simulink model "example_sdofplant"  (R2024b)
settings: Solver=FixedStepAuto  StartTime=0  StopTime=200  FixedStep=5/1000  RelTol=1e-3
model workspace (MAT data in the model file):
  Sig : Simulink.Signal (value not decoded)
  Sig1 : Simulink.Signal (value not decoded)
  Sig2 : Simulink.Signal (value not decoded)
  Sig3 : Simulink.Signal (value not decoded)
  Sig4 : Simulink.Signal (value not decoded)
  Sig5 : Simulink.Signal (value not decoded)
  Sig6 : Simulink.Signal (value not decoded)
values from neighbouring files (symbols this model uses):
  aerody =     [vtol50kg_airframe_data.mat]    (also in vtol50kg_airframe_init.m = init_aerody; vtol50kg_initdata.m = init_aerody)
  engine =     [vtol50kg_airframe_data.mat]    (also in vtol50kg_airframe_init.m = init_engine; vtol50kg_initdata.m = init_engine)
  mass =     [vtol50kg_airframe_data.mat]    (also in vtol50kg_airframe_init.m = init_weight; vtol50kg_initdata.m = init_weight)
  motor =     [vtol50kg_airframe_data.mat]    (also in vtol50kg_airframe_init.m = init_motor; vtol50kg_initdata.m = init_motor)
undefined symbols (not defined in the file or in its folder): convertTo, datetime, Earth, F, Light, MIL, plant, WGS84, WMM2020
libraries: aerolibconvert2 x5, aerolibasang x5, aerolibwind2 x3, aerolibactuator x2, shared6dof x1, aerolibatmos2 x1, aerolibtransform2 x1, aerolibgravity2 x1
(part 2 of 2)

== system example_sdofplant/state/Variant Subsystem/Subsystem1 ==
  h(m) : Inport
  μ(deg) : Inport  Port=2
  l(deg) : Inport  Port=3
  World Magnetic Model : aerolibgravity2/World Magnetic Model  model=WMM2020 (2020-2025)  customFile='WMM2020.COF'  units=Metric (MKS)  time_in=off  month=January  day=1  year=2020  action=Error  h_out=on  dec_out=on  inc_out=on  ti_out=on
  XYZ(nT) : Outport
  H(nT) : Outport  Port=2
  D(deg) : Outport  Port=3
  I(deg) : Outport  Port=4
  F(nT) : Outport  Port=5
  wires:
  h(m)/1 -> World Magnetic Model/1
  World Magnetic Model/1 -> XYZ(nT)/1
  World Magnetic Model/2 -> H(nT)/1
  World Magnetic Model/3 -> D(deg)/1
  World Magnetic Model/4 -> I(deg)/1
  World Magnetic Model/5 -> F(nT)/1
  l(deg)/1 -> World Magnetic Model/3
  μ(deg)/1 -> World Magnetic Model/2

== system example_sdofplant/actuator/fixed wing/actuator dyanmics/Variant Subsystem ==
  note: 1) Add Subsystem or Model blocks as valid variant choices.
      | 2) You cannot connect blocks at this level. At simulation, connectivity is automatically
      | determined, based on the active variant and port name matching.
  In1 : Inport
  Subsystem : Subsystem  VariantControl=true
  Subsystem1 : Subsystem  VariantControl=false
  Out1 : Outport

== system example_sdofplant/actuator/fixed wing/aerodynamics/basic ==
  alpha : Inport  Unit=deg
  beta : Inport  Port=2  Unit=deg
  2-D Lookup Table : Lookup_n-D  LookupTableObject=''  BreakpointsForDimension1=aerody.basic.cx.alpha  BreakpointsForDimension2=aerody.basic.cx.beta  BreakpointsForDimension1FirstPoint=10  BreakpointsForDimension2FirstPoint=10  BreakpointsForDimension1Spacing=12  BreakpointsForDimension2Spacing=12  IndexSearchMethod=Linear search  BeginIndexSearchUsingPreviousIndexResult=on  Table=aerody.basic.cx.coeff  ExtrapMethod=Clip  DiagnosticForOutOfRangeInput=Warning  InternalRulePriority=Speed  RndMeth=Simplest
      settings: InputPortMap=u0,u1
  2-D Lookup Table1 : Lookup_n-D  LookupTableObject=''  BreakpointsForDimension1=aerody.basic.cy.alpha  BreakpointsForDimension2=aerody.basic.cy.beta  BreakpointsForDimension1FirstPoint=10  BreakpointsForDimension2FirstPoint=10  BreakpointsForDimension1Spacing=12  BreakpointsForDimension2Spacing=12  IndexSearchMethod=Linear search  BeginIndexSearchUsingPreviousIndexResult=on  Table=aerody.basic.cy.coeff  ExtrapMethod=Clip  DiagnosticForOutOfRangeInput=Warning  InternalRulePriority=Speed  RndMeth=Simplest
      settings: InputPortMap=u0,u1
  2-D Lookup Table2 : Lookup_n-D  LookupTableObject=''  BreakpointsForDimension1=aerody.basic.cz.alpha  BreakpointsForDimension2=aerody.basic.cz.beta  BreakpointsForDimension1FirstPoint=10  BreakpointsForDimension2FirstPoint=10  BreakpointsForDimension1Spacing=12  BreakpointsForDimension2Spacing=12  IndexSearchMethod=Linear search  BeginIndexSearchUsingPreviousIndexResult=on  Table=aerody.basic.cz.coeff  ExtrapMethod=Clip  DiagnosticForOutOfRangeInput=Warning  InternalRulePriority=Speed  RndMeth=Simplest
      settings: InputPortMap=u0,u1
  2-D Lookup Table3 : Lookup_n-D  LookupTableObject=''  BreakpointsForDimension1=aerody.basic.cll.alpha  BreakpointsForDimension2=aerody.basic.cll.beta  BreakpointsForDimension1FirstPoint=10  BreakpointsForDimension2FirstPoint=10  BreakpointsForDimension1Spacing=12  BreakpointsForDimension2Spacing=12  IndexSearchMethod=Linear search  BeginIndexSearchUsingPreviousIndexResult=on  Table=aerody.basic.cll.coeff  ExtrapMethod=Clip  DiagnosticForOutOfRangeInput=Warning  InternalRulePriority=Speed  RndMeth=Simplest
      settings: InputPortMap=u0,u1
  2-D Lookup Table4 : Lookup_n-D  LookupTableObject=''  BreakpointsForDimension1=aerody.basic.cm.alpha  BreakpointsForDimension2=aerody.basic.cm.beta  BreakpointsForDimension1FirstPoint=10  BreakpointsForDimension2FirstPoint=10  BreakpointsForDimension1Spacing=12  BreakpointsForDimension2Spacing=12  IndexSearchMethod=Linear search  BeginIndexSearchUsingPreviousIndexResult=on  Table=aerody.basic.cm.coeff  ExtrapMethod=Clip  DiagnosticForOutOfRangeInput=Warning  InternalRulePriority=Speed  RndMeth=Simplest
      settings: InputPortMap=u0,u1
  2-D Lookup Table5 : Lookup_n-D  LookupTableObject=''  BreakpointsForDimension1=aerody.basic.cn.alpha  BreakpointsForDimension2=aerody.basic.cn.beta  BreakpointsForDimension1FirstPoint=10  BreakpointsForDimension2FirstPoint=10  BreakpointsForDimension1Spacing=12  BreakpointsForDimension2Spacing=12  IndexSearchMethod=Linear search  BeginIndexSearchUsingPreviousIndexResult=on  Table=aerody.basic.cn.coeff  ExtrapMethod=Clip  DiagnosticForOutOfRangeInput=Warning  InternalRulePriority=Speed  RndMeth=Simplest
      settings: InputPortMap=u0,u1
  Mux : Mux  Inputs=3
  Mux1 : Mux  Inputs=3
  cxcycz : Outport
  clcmcn : Outport  Port=2
  wires:
  alpha/1 -> 2-D Lookup Table5/1, 2-D Lookup Table4/1, 2-D Lookup Table3/1, 2-D Lookup Table2/1, 2-D Lookup Table1/1, 2-D Lookup Table/1
  beta/1 -> 2-D Lookup Table/2, 2-D Lookup Table5/2, 2-D Lookup Table4/2, 2-D Lookup Table3/2, 2-D Lookup Table2/2, 2-D Lookup Table1/2
  2-D Lookup Table/1 -> Mux/1
  Mux/1 -> cxcycz/1
  2-D Lookup Table1/1 -> Mux/2
  2-D Lookup Table2/1 -> Mux/3
  2-D Lookup Table5/1 -> Mux1/3
  2-D Lookup Table4/1 -> Mux1/2
  Mux1/1 -> clcmcn/1
  2-D Lookup Table3/1 -> Mux1/1

== system example_sdofplant/actuator/fixed wing/aerodynamics/landgear ==
  alpha : Inport
  beta : Inport  Port=2
  2-D Lookup Table : Lookup_n-D  LookupTableObject=''  BreakpointsForDimension1=aerody.landgear.cx.alpha  BreakpointsForDimension2=aerody.landgear.cx.beta  BreakpointsForDimension1FirstPoint=10  BreakpointsForDimension2FirstPoint=10  BreakpointsForDimension1Spacing=12  BreakpointsForDimension2Spacing=12  IndexSearchMethod=Linear search  BeginIndexSearchUsingPreviousIndexResult=on  Table=aerody.landgear.cx.coeff  ExtrapMethod=Clip  DiagnosticForOutOfRangeInput=Warning  InternalRulePriority=Speed  RndMeth=Simplest
      settings: InputPortMap=u0,u1
  2-D Lookup Table1 : Lookup_n-D  LookupTableObject=''  BreakpointsForDimension1=aerody.landgear.cy.alpha  BreakpointsForDimension2=aerody.landgear.cy.beta  BreakpointsForDimension1FirstPoint=10  BreakpointsForDimension2FirstPoint=10  BreakpointsForDimension1Spacing=12  BreakpointsForDimension2Spacing=12  IndexSearchMethod=Linear search  BeginIndexSearchUsingPreviousIndexResult=on  Table=aerody.landgear.cy.coeff  ExtrapMethod=Clip  DiagnosticForOutOfRangeInput=Warning  InternalRulePriority=Speed  RndMeth=Simplest
      settings: InputPortMap=u0,u1
  2-D Lookup Table2 : Lookup_n-D  LookupTableObject=''  BreakpointsForDimension1=aerody.landgear.cz.alpha  BreakpointsForDimension2=aerody.landgear.cz.beta  BreakpointsForDimension1FirstPoint=10  BreakpointsForDimension2FirstPoint=10  BreakpointsForDimension1Spacing=12  BreakpointsForDimension2Spacing=12  IndexSearchMethod=Linear search  BeginIndexSearchUsingPreviousIndexResult=on  Table=aerody.landgear.cz.coeff  ExtrapMethod=Clip  DiagnosticForOutOfRangeInput=Warning  InternalRulePriority=Speed  RndMeth=Simplest
      settings: InputPortMap=u0,u1
  2-D Lookup Table3 : Lookup_n-D  LookupTableObject=''  BreakpointsForDimension1=aerody.landgear.cll.alpha  BreakpointsForDimension2=aerody.landgear.cll.beta  BreakpointsForDimension1FirstPoint=10  BreakpointsForDimension2FirstPoint=10  BreakpointsForDimension1Spacing=12  BreakpointsForDimension2Spacing=12  IndexSearchMethod=Linear search  BeginIndexSearchUsingPreviousIndexResult=on  Table=aerody.landgear.cll.coeff  ExtrapMethod=Clip  DiagnosticForOutOfRangeInput=Warning  InternalRulePriority=Speed  RndMeth=Simplest
      settings: InputPortMap=u0,u1
  2-D Lookup Table4 : Lookup_n-D  LookupTableObject=''  BreakpointsForDimension1=aerody.landgear.cm.alpha  BreakpointsForDimension2=aerody.landgear.cm.beta  BreakpointsForDimension1FirstPoint=10  BreakpointsForDimension2FirstPoint=10  BreakpointsForDimension1Spacing=12  BreakpointsForDimension2Spacing=12  IndexSearchMethod=Linear search  BeginIndexSearchUsingPreviousIndexResult=on  Table=aerody.landgear.cm.coeff  ExtrapMethod=Clip  DiagnosticForOutOfRangeInput=Warning  InternalRulePriority=Speed  RndMeth=Simplest
      settings: InputPortMap=u0,u1
  2-D Lookup Table5 : Lookup_n-D  LookupTableObject=''  BreakpointsForDimension1=aerody.landgear.cn.alpha  BreakpointsForDimension2=aerody.landgear.cn.beta  BreakpointsForDimension1FirstPoint=10  BreakpointsForDimension2FirstPoint=10  BreakpointsForDimension1Spacing=12  BreakpointsForDimension2Spacing=12  IndexSearchMethod=Linear search  BeginIndexSearchUsingPreviousIndexResult=on  Table=aerody.landgear.cn.coeff  ExtrapMethod=Clip  DiagnosticForOutOfRangeInput=Warning  InternalRulePriority=Speed  RndMeth=Simplest
      settings: InputPortMap=u0,u1
  Mux : Mux  Inputs=3
  Mux1 : Mux  Inputs=3
  cxcycz : Outport
  clcmcn : Outport  Port=2
  wires:
  alpha/1 -> 2-D Lookup Table5/1, 2-D Lookup Table4/1, 2-D Lookup Table3/1, 2-D Lookup Table2/1, 2-D Lookup Table1/1, 2-D Lookup Table/1
  beta/1 -> 2-D Lookup Table/2, 2-D Lookup Table5/2, 2-D Lookup Table4/2, 2-D Lookup Table3/2, 2-D Lookup Table2/2, 2-D Lookup Table1/2
  2-D Lookup Table/1 -> Mux/1
  Mux/1 -> cxcycz/1
  2-D Lookup Table1/1 -> Mux/2
  2-D Lookup Table2/1 -> Mux/3
  Mux1/1 -> clcmcn/1
  2-D Lookup Table3/1 -> Mux1/1
  2-D Lookup Table4/1 -> Mux1/2
  2-D Lookup Table5/1 -> Mux1/3

== system example_sdofplant/actuator/fixed wing/aerodynamics/left aileron ==
  alpha : Inport
  beta : Inport  Port=2
  dla : Inport  Port=3
  2-D Lookup Table : Lookup_n-D  NumberOfTableDimensions=3  LookupTableObject=''  BreakpointsForDimension1=aerody.left_aileron.cx.alpha  BreakpointsForDimension2=aerody.left_aileron.cx.beta  BreakpointsForDimension3=aerody.left_aileron.cx.delta  BreakpointsForDimension1FirstPoint=10  BreakpointsForDimension2FirstPoint=10  BreakpointsForDimension1Spacing=12  BreakpointsForDimension2Spacing=12  IndexSearchMethod=Linear search  BeginIndexSearchUsingPreviousIndexResult=on  Table=aerody.left_aileron.cx.coeff  ExtrapMethod=Clip  DiagnosticForOutOfRangeInput=Warning  InternalRulePriority=Speed  RndMeth=Simplest
      settings: InputPortMap=u0,u1,u2
  2-D Lookup Table1 : Lookup_n-D  NumberOfTableDimensions=3  LookupTableObject=''  BreakpointsForDimension1=aerody.left_aileron.cz.alpha  BreakpointsForDimension2=aerody.left_aileron.cz.beta  BreakpointsForDimension3=aerody.left_aileron.cz.delta  BreakpointsForDimension1FirstPoint=10  BreakpointsForDimension2FirstPoint=10  BreakpointsForDimension1Spacing=12  BreakpointsForDimension2Spacing=12  IndexSearchMethod=Linear search  BeginIndexSearchUsingPreviousIndexResult=on  Table=aerody.left_aileron.cz.coeff  ExtrapMethod=Clip  DiagnosticForOutOfRangeInput=Warning  InternalRulePriority=Speed  RndMeth=Simplest
      settings: InputPortMap=u0,u1,u2
  2-D Lookup Table2 : Lookup_n-D  NumberOfTableDimensions=3  LookupTableObject=''  BreakpointsForDimension1=aerody.left_aileron.cll.alpha  BreakpointsForDimension2=aerody.left_aileron.cll.beta  BreakpointsForDimension3=aerody.left_aileron.cll.delta  BreakpointsForDimension1FirstPoint=10  BreakpointsForDimension2FirstPoint=10  BreakpointsForDimension1Spacing=12  BreakpointsForDimension2Spacing=12  IndexSearchMethod=Linear search  BeginIndexSearchUsingPreviousIndexResult=on  Table=aerody.left_aileron.cll.coeff  ExtrapMethod=Clip  DiagnosticForOutOfRangeInput=Warning  InternalRulePriority=Speed  RndMeth=Simplest
      settings: InputPortMap=u0,u1,u2
  2-D Lookup Table3 : Lookup_n-D  NumberOfTableDimensions=3  LookupTableObject=''  BreakpointsForDimension1=aerody.left_aileron.cm.alpha  BreakpointsForDimension2=aerody.left_aileron.cm.beta  BreakpointsForDimension3=aerody.left_aileron.cm.delta  BreakpointsForDimension1FirstPoint=10  BreakpointsForDimension2FirstPoint=10  BreakpointsForDimension1Spacing=12  BreakpointsForDimension2Spacing=12  IndexSearchMethod=Linear search  BeginIndexSearchUsingPreviousIndexResult=on  Table=aerody.left_aileron.cm.coeff  ExtrapMethod=Clip  DiagnosticForOutOfRangeInput=Warning  InternalRulePriority=Speed  RndMeth=Simplest
      settings: InputPortMap=u0,u1,u2
  2-D Lookup Table4 : Lookup_n-D  NumberOfTableDimensions=3  LookupTableObject=''  BreakpointsForDimension1=aerody.left_aileron.cn.alpha  BreakpointsForDimension2=aerody.left_aileron.cn.beta  BreakpointsForDimension3=aerody.left_aileron.cn.delta  BreakpointsForDimension1FirstPoint=10  BreakpointsForDimension2FirstPoint=10  BreakpointsForDimension1Spacing=12  BreakpointsForDimension2Spacing=12  IndexSearchMethod=Linear search  BeginIndexSearchUsingPreviousIndexResult=on  Table=aerody.left_aileron.cn.coeff  ExtrapMethod=Clip  DiagnosticForOutOfRangeInput=Warning  InternalRulePriority=Speed  RndMeth=Simplest
      settings: InputPortMap=u0,u1,u2
  2-D Lookup Table6 : Lookup_n-D  NumberOfTableDimensions=3  LookupTableObject=''  BreakpointsForDimension1=aerody.left_aileron.cy.alpha  BreakpointsForDimension2=aerody.left_aileron.cy.beta  BreakpointsForDimension3=aerody.left_aileron.cy.delta  BreakpointsForDimension1FirstPoint=10  BreakpointsForDimension2FirstPoint=10  BreakpointsForDimension1Spacing=12  BreakpointsForDimension2Spacing=12  IndexSearchMethod=Linear search  BeginIndexSearchUsingPreviousIndexResult=on  Table=aerody.left_aileron.cy.coeff  ExtrapMethod=Clip  DiagnosticForOutOfRangeInput=Warning  InternalRulePriority=Speed  RndMeth=Simplest
      settings: InputPortMap=u0,u1,u2
  Mux : Mux  Inputs=3
  Mux1 : Mux  Inputs=3
  cxcycz : Outport
  clcmcn : Outport  Port=2
  wires:
  2-D Lookup Table1/1 -> Mux/3
  2-D Lookup Table/1 -> Mux/1
  Mux/1 -> cxcycz/1
  Mux1/1 -> clcmcn/1
  2-D Lookup Table6/1 -> Mux/2
  alpha/1 -> 2-D Lookup Table6/1, 2-D Lookup Table1/1, 2-D Lookup Table2/1, 2-D Lookup Table4/1, 2-D Lookup Table3/1, 2-D Lookup Table/1
  beta/1 -> 2-D Lookup Table6/2, 2-D Lookup Table1/2, 2-D Lookup Table2/2, 2-D Lookup Table4/2, 2-D Lookup Table3/2, 2-D Lookup Table/2
  dla/1 -> 2-D Lookup Table/3, 2-D Lookup Table6/3, 2-D Lookup Table1/3, 2-D Lookup Table2/3, 2-D Lookup Table4/3, 2-D Lookup Table3/3
  2-D Lookup Table2/1 -> Mux1/1
  2-D Lookup Table3/1 -> Mux1/2
  2-D Lookup Table4/1 -> Mux1/3

== system example_sdofplant/actuator/fixed wing/aerodynamics/left rudder ==
  alpha : Inport
  beta : Inport  Port=2
  dlr : Inport  Port=3
  2-D Lookup Table : Lookup_n-D  NumberOfTableDimensions=3  LookupTableObject=''  BreakpointsForDimension1=aerody.left_rudder.cx.alpha  BreakpointsForDimension2=aerody.left_rudder.cx.beta  BreakpointsForDimension3=aerody.left_rudder.cx.delta  BreakpointsForDimension1FirstPoint=10  BreakpointsForDimension2FirstPoint=10  BreakpointsForDimension1Spacing=12  BreakpointsForDimension2Spacing=12  IndexSearchMethod=Linear search  BeginIndexSearchUsingPreviousIndexResult=on  Table=aerody.left_rudder.cx.coeff  ExtrapMethod=Clip  DiagnosticForOutOfRangeInput=Warning  InternalRulePriority=Speed  RndMeth=Simplest
      settings: InputPortMap=u0,u1,u2
  2-D Lookup Table1 : Lookup_n-D  NumberOfTableDimensions=3  LookupTableObject=''  BreakpointsForDimension1=aerody.left_rudder.cy.alpha  BreakpointsForDimension2=aerody.left_rudder.cy.beta  BreakpointsForDimension3=aerody.left_rudder.cy.delta  BreakpointsForDimension1FirstPoint=10  BreakpointsForDimension2FirstPoint=10  BreakpointsForDimension1Spacing=12  BreakpointsForDimension2Spacing=12  IndexSearchMethod=Linear search  BeginIndexSearchUsingPreviousIndexResult=on  Table=aerody.left_rudder.cy.coeff  ExtrapMethod=Clip  DiagnosticForOutOfRangeInput=Warning  InternalRulePriority=Speed  RndMeth=Simplest
      settings: InputPortMap=u0,u1,u2
  2-D Lookup Table2 : Lookup_n-D  NumberOfTableDimensions=3  LookupTableObject=''  BreakpointsForDimension1=aerody.left_rudder.cz.alpha  BreakpointsForDimension2=aerody.left_rudder.cz.beta  BreakpointsForDimension3=aerody.left_rudder.cz.delta  BreakpointsForDimension1FirstPoint=10  BreakpointsForDimension2FirstPoint=10  BreakpointsForDimension1Spacing=12  BreakpointsForDimension2Spacing=12  IndexSearchMethod=Linear search  BeginIndexSearchUsingPreviousIndexResult=on  Table=aerody.left_rudder.cz.coeff  ExtrapMethod=Clip  DiagnosticForOutOfRangeInput=Warning  InternalRulePriority=Speed  RndMeth=Simplest
      settings: InputPortMap=u0,u1,u2
  2-D Lookup Table3 : Lookup_n-D  NumberOfTableDimensions=3  LookupTableObject=''  BreakpointsForDimension1=aerody.left_rudder.cll.alpha  BreakpointsForDimension2=aerody.left_rudder.cll.beta  BreakpointsForDimension3=aerody.left_rudder.cll.delta  BreakpointsForDimension1FirstPoint=10  BreakpointsForDimension2FirstPoint=10  BreakpointsForDimension1Spacing=12  BreakpointsForDimension2Spacing=12  IndexSearchMethod=Linear search  BeginIndexSearchUsingPreviousIndexResult=on  Table=aerody.left_rudder.cll.coeff  ExtrapMethod=Clip  DiagnosticForOutOfRangeInput=Warning  InternalRulePriority=Speed  RndMeth=Simplest
      settings: InputPortMap=u0,u1,u2
  2-D Lookup Table4 : Lookup_n-D  NumberOfTableDimensions=3  LookupTableObject=''  BreakpointsForDimension1=aerody.left_rudder.cm.alpha  BreakpointsForDimension2=aerody.left_rudder.cm.beta  BreakpointsForDimension3=aerody.left_rudder.cm.delta  BreakpointsForDimension1FirstPoint=10  BreakpointsForDimension2FirstPoint=10  BreakpointsForDimension1Spacing=12  BreakpointsForDimension2Spacing=12  IndexSearchMethod=Linear search  BeginIndexSearchUsingPreviousIndexResult=on  Table=aerody.left_rudder.cm.coeff  ExtrapMethod=Clip  DiagnosticForOutOfRangeInput=Warning  InternalRulePriority=Speed  RndMeth=Simplest
      settings: InputPortMap=u0,u1,u2
  2-D Lookup Table5 : Lookup_n-D  NumberOfTableDimensions=3  LookupTableObject=''  BreakpointsForDimension1=aerody.left_rudder.cn.alpha  BreakpointsForDimension2=aerody.left_rudder.cn.beta  BreakpointsForDimension3=aerody.left_rudder.cn.delta  BreakpointsForDimension1FirstPoint=10  BreakpointsForDimension2FirstPoint=10  BreakpointsForDimension1Spacing=12  BreakpointsForDimension2Spacing=12  IndexSearchMethod=Linear search  BeginIndexSearchUsingPreviousIndexResult=on  Table=aerody.left_rudder.cn.coeff  ExtrapMethod=Clip  DiagnosticForOutOfRangeInput=Warning  InternalRulePriority=Speed  RndMeth=Simplest
      settings: InputPortMap=u0,u1,u2
  Mux : Mux  Inputs=3
  Mux1 : Mux  Inputs=3
  cxcycz : Outport
  clcmcn : Outport  Port=2
  wires:
  2-D Lookup Table/1 -> Mux/1
  2-D Lookup Table1/1 -> Mux/2
  Mux/1 -> cxcycz/1
  Mux1/1 -> clcmcn/1
  2-D Lookup Table2/1 -> Mux/3
  dlr/1 -> 2-D Lookup Table1/3, 2-D Lookup Table/3, 2-D Lookup Table2/3, 2-D Lookup Table3/3, 2-D Lookup Table5/3, 2-D Lookup Table4/3
  beta/1 -> 2-D Lookup Table/2, 2-D Lookup Table1/2, 2-D Lookup Table2/2, 2-D Lookup Table3/2, 2-D Lookup Table5/2, 2-D Lookup Table4/2
  alpha/1 -> 2-D Lookup Table/1, 2-D Lookup Table1/1, 2-D Lookup Table2/1, 2-D Lookup Table3/1, 2-D Lookup Table5/1, 2-D Lookup Table4/1
  2-D Lookup Table3/1 -> Mux1/1
  2-D Lookup Table4/1 -> Mux1/2
  2-D Lookup Table5/1 -> Mux1/3

== system example_sdofplant/actuator/fixed wing/aerodynamics/right aileron ==
  alpha : Inport
  beta : Inport  Port=2
  dra : Inport  Port=3
  2-D Lookup Table : Lookup_n-D  NumberOfTableDimensions=3  LookupTableObject=''  BreakpointsForDimension1=aerody.right_aileron.cx.alpha  BreakpointsForDimension2=aerody.right_aileron.cx.beta  BreakpointsForDimension3=aerody.right_aileron.cx.delta  BreakpointsForDimension1FirstPoint=10  BreakpointsForDimension2FirstPoint=10  BreakpointsForDimension1Spacing=12  BreakpointsForDimension2Spacing=12  IndexSearchMethod=Linear search  BeginIndexSearchUsingPreviousIndexResult=on  Table=aerody.right_aileron.cx.coeff  ExtrapMethod=Clip  DiagnosticForOutOfRangeInput=Warning  InternalRulePriority=Speed  RndMeth=Simplest
      settings: InputPortMap=u0,u1,u2
  2-D Lookup Table1 : Lookup_n-D  NumberOfTableDimensions=3  LookupTableObject=''  BreakpointsForDimension1=aerody.right_aileron.cy.alpha  BreakpointsForDimension2=aerody.right_aileron.cy.beta  BreakpointsForDimension3=aerody.right_aileron.cy.delta  BreakpointsForDimension1FirstPoint=10  BreakpointsForDimension2FirstPoint=10  BreakpointsForDimension1Spacing=12  BreakpointsForDimension2Spacing=12  IndexSearchMethod=Linear search  BeginIndexSearchUsingPreviousIndexResult=on  Table=aerody.right_aileron.cy.coeff  ExtrapMethod=Clip  DiagnosticForOutOfRangeInput=Warning  InternalRulePriority=Speed  RndMeth=Simplest
      settings: InputPortMap=u0,u1,u2
  2-D Lookup Table2 : Lookup_n-D  NumberOfTableDimensions=3  LookupTableObject=''  BreakpointsForDimension1=aerody.right_aileron.cz.alpha  BreakpointsForDimension2=aerody.right_aileron.cz.beta  BreakpointsForDimension3=aerody.right_aileron.cz.delta  BreakpointsForDimension1FirstPoint=10  BreakpointsForDimension2FirstPoint=10  BreakpointsForDimension1Spacing=12  BreakpointsForDimension2Spacing=12  IndexSearchMethod=Linear search  BeginIndexSearchUsingPreviousIndexResult=on  Table=aerody.right_aileron.cz.coeff  ExtrapMethod=Clip  DiagnosticForOutOfRangeInput=Warning  InternalRulePriority=Speed  RndMeth=Simplest
      settings: InputPortMap=u0,u1,u2
  2-D Lookup Table3 : Lookup_n-D  NumberOfTableDimensions=3  LookupTableObject=''  BreakpointsForDimension1=aerody.right_aileron.cll.alpha  BreakpointsForDimension2=aerody.right_aileron.cll.beta  BreakpointsForDimension3=aerody.right_aileron.cll.delta  BreakpointsForDimension1FirstPoint=10  BreakpointsForDimension2FirstPoint=10  BreakpointsForDimension1Spacing=12  BreakpointsForDimension2Spacing=12  IndexSearchMethod=Linear search  BeginIndexSearchUsingPreviousIndexResult=on  Table=aerody.right_aileron.cll.coeff  ExtrapMethod=Clip  DiagnosticForOutOfRangeInput=Warning  InternalRulePriority=Speed  RndMeth=Simplest
      settings: InputPortMap=u0,u1,u2
  2-D Lookup Table4 : Lookup_n-D  NumberOfTableDimensions=3  LookupTableObject=''  BreakpointsForDimension1=aerody.right_aileron.cm.alpha  BreakpointsForDimension2=aerody.right_aileron.cm.beta  BreakpointsForDimension3=aerody.right_aileron.cm.delta  BreakpointsForDimension1FirstPoint=10  BreakpointsForDimension2FirstPoint=10  BreakpointsForDimension1Spacing=12  BreakpointsForDimension2Spacing=12  IndexSearchMethod=Linear search  BeginIndexSearchUsingPreviousIndexResult=on  Table=aerody.right_aileron.cm.coeff  ExtrapMethod=Clip  DiagnosticForOutOfRangeInput=Warning  InternalRulePriority=Speed  RndMeth=Simplest
      settings: InputPortMap=u0,u1,u2
  2-D Lookup Table5 : Lookup_n-D  NumberOfTableDimensions=3  LookupTableObject=''  BreakpointsForDimension1=aerody.right_aileron.cn.alpha  BreakpointsForDimension2=aerody.right_aileron.cn.beta  BreakpointsForDimension3=aerody.right_aileron.cn.delta  BreakpointsForDimension1FirstPoint=10  BreakpointsForDimension2FirstPoint=10  BreakpointsForDimension1Spacing=12  BreakpointsForDimension2Spacing=12  IndexSearchMethod=Linear search  BeginIndexSearchUsingPreviousIndexResult=on  Table=aerody.right_aileron.cn.coeff  ExtrapMethod=Clip  DiagnosticForOutOfRangeInput=Warning  InternalRulePriority=Speed  RndMeth=Simplest
      settings: InputPortMap=u0,u1,u2
  Mux : Mux  Inputs=3
  Mux1 : Mux  Inputs=3
  cxcycz : Outport
  clcmcn : Outport  Port=2
  wires:
  2-D Lookup Table/1 -> Mux/1
  2-D Lookup Table1/1 -> Mux/2
  Mux/1 -> cxcycz/1
  Mux1/1 -> clcmcn/1
  2-D Lookup Table2/1 -> Mux/3
  beta/1 -> 2-D Lookup Table/2, 2-D Lookup Table1/2, 2-D Lookup Table2/2, 2-D Lookup Table3/2, 2-D Lookup Table5/2, 2-D Lookup Table4/2
  dra/1 -> 2-D Lookup Table1/3, 2-D Lookup Table/3, 2-D Lookup Table2/3, 2-D Lookup Table3/3, 2-D Lookup Table5/3, 2-D Lookup Table4/3
  alpha/1 -> 2-D Lookup Table/1, 2-D Lookup Table1/1, 2-D Lookup Table2/1, 2-D Lookup Table3/1, 2-D Lookup Table5/1, 2-D Lookup Table4/1
  2-D Lookup Table3/1 -> Mux1/1
  2-D Lookup Table4/1 -> Mux1/2
  2-D Lookup Table5/1 -> Mux1/3

== system example_sdofplant/actuator/fixed wing/aerodynamics/right rudder ==
  alpha : Inport
  beta : Inport  Port=2
  drr : Inport  Port=3
  2-D Lookup Table : Lookup_n-D  NumberOfTableDimensions=3  LookupTableObject=''  BreakpointsForDimension1=aerody.right_rudder.cx.alpha  BreakpointsForDimension2=aerody.right_rudder.cx.beta  BreakpointsForDimension3=aerody.right_rudder.cx.delta  BreakpointsForDimension1FirstPoint=10  BreakpointsForDimension2FirstPoint=10  BreakpointsForDimension1Spacing=12  BreakpointsForDimension2Spacing=12  IndexSearchMethod=Linear search  BeginIndexSearchUsingPreviousIndexResult=on  Table=aerody.right_rudder.cx.coeff  ExtrapMethod=Clip  DiagnosticForOutOfRangeInput=Warning  InternalRulePriority=Speed  RndMeth=Simplest
      settings: InputPortMap=u0,u1,u2
  2-D Lookup Table1 : Lookup_n-D  NumberOfTableDimensions=3  LookupTableObject=''  BreakpointsForDimension1=aerody.right_rudder.cy.alpha  BreakpointsForDimension2=aerody.right_rudder.cy.beta  BreakpointsForDimension3=aerody.right_rudder.cy.delta  BreakpointsForDimension1FirstPoint=10  BreakpointsForDimension2FirstPoint=10  BreakpointsForDimension1Spacing=12  BreakpointsForDimension2Spacing=12  IndexSearchMethod=Linear search  BeginIndexSearchUsingPreviousIndexResult=on  Table=aerody.right_rudder.cy.coeff  ExtrapMethod=Clip  DiagnosticForOutOfRangeInput=Warning  InternalRulePriority=Speed  RndMeth=Simplest
      settings: InputPortMap=u0,u1,u2
  2-D Lookup Table2 : Lookup_n-D  NumberOfTableDimensions=3  LookupTableObject=''  BreakpointsForDimension1=aerody.right_rudder.cz.alpha  BreakpointsForDimension2=aerody.right_rudder.cz.beta  BreakpointsForDimension3=aerody.right_rudder.cz.delta  BreakpointsForDimension1FirstPoint=10  BreakpointsForDimension2FirstPoint=10  BreakpointsForDimension1Spacing=12  BreakpointsForDimension2Spacing=12  IndexSearchMethod=Linear search  BeginIndexSearchUsingPreviousIndexResult=on  Table=aerody.right_rudder.cz.coeff  ExtrapMethod=Clip  DiagnosticForOutOfRangeInput=Warning  InternalRulePriority=Speed  RndMeth=Simplest
      settings: InputPortMap=u0,u1,u2
  2-D Lookup Table3 : Lookup_n-D  NumberOfTableDimensions=3  LookupTableObject=''  BreakpointsForDimension1=aerody.right_rudder.cll.alpha  BreakpointsForDimension2=aerody.right_rudder.cll.beta  BreakpointsForDimension3=aerody.right_rudder.cll.delta  BreakpointsForDimension1FirstPoint=10  BreakpointsForDimension2FirstPoint=10  BreakpointsForDimension1Spacing=12  BreakpointsForDimension2Spacing=12  IndexSearchMethod=Linear search  BeginIndexSearchUsingPreviousIndexResult=on  Table=aerody.right_rudder.cll.coeff  ExtrapMethod=Clip  DiagnosticForOutOfRangeInput=Warning  InternalRulePriority=Speed  RndMeth=Simplest
      settings: InputPortMap=u0,u1,u2
  2-D Lookup Table4 : Lookup_n-D  NumberOfTableDimensions=3  LookupTableObject=''  BreakpointsForDimension1=aerody.right_rudder.cm.alpha  BreakpointsForDimension2=aerody.right_rudder.cm.beta  BreakpointsForDimension3=aerody.right_rudder.cm.delta  BreakpointsForDimension1FirstPoint=10  BreakpointsForDimension2FirstPoint=10  BreakpointsForDimension1Spacing=12  BreakpointsForDimension2Spacing=12  IndexSearchMethod=Linear search  BeginIndexSearchUsingPreviousIndexResult=on  Table=aerody.right_rudder.cm.coeff  ExtrapMethod=Clip  DiagnosticForOutOfRangeInput=Warning  InternalRulePriority=Speed  RndMeth=Simplest
      settings: InputPortMap=u0,u1,u2
  2-D Lookup Table5 : Lookup_n-D  NumberOfTableDimensions=3  LookupTableObject=''  BreakpointsForDimension1=aerody.right_rudder.cn.alpha  BreakpointsForDimension2=aerody.right_rudder.cn.beta  BreakpointsForDimension3=aerody.right_rudder.cn.delta  BreakpointsForDimension1FirstPoint=10  BreakpointsForDimension2FirstPoint=10  BreakpointsForDimension1Spacing=12  BreakpointsForDimension2Spacing=12  IndexSearchMethod=Linear search  BeginIndexSearchUsingPreviousIndexResult=on  Table=aerody.right_rudder.cn.coeff  ExtrapMethod=Clip  DiagnosticForOutOfRangeInput=Warning  InternalRulePriority=Speed  RndMeth=Simplest
      settings: InputPortMap=u0,u1,u2
  Mux : Mux  Inputs=3
  Mux1 : Mux  Inputs=3
  cxcycz : Outport
  clcmcn : Outport  Port=2
  wires:
  2-D Lookup Table/1 -> Mux/1
  2-D Lookup Table1/1 -> Mux/2
  Mux/1 -> cxcycz/1
  Mux1/1 -> clcmcn/1
  2-D Lookup Table2/1 -> Mux/3
  drr/1 -> 2-D Lookup Table/3, 2-D Lookup Table1/3, 2-D Lookup Table2/3, 2-D Lookup Table3/3, 2-D Lookup Table5/3, 2-D Lookup Table4/3
  beta/1 -> 2-D Lookup Table/2, 2-D Lookup Table1/2, 2-D Lookup Table2/2, 2-D Lookup Table3/2, 2-D Lookup Table5/2, 2-D Lookup Table4/2
  alpha/1 -> 2-D Lookup Table/1, 2-D Lookup Table1/1, 2-D Lookup Table2/1, 2-D Lookup Table3/1, 2-D Lookup Table5/1, 2-D Lookup Table4/1
  2-D Lookup Table3/1 -> Mux1/1
  2-D Lookup Table4/1 -> Mux1/2
  2-D Lookup Table5/1 -> Mux1/3

== system example_sdofplant/actuator/fixed wing/actuator dyanmics/Variant Subsystem/Subsystem ==
  In1 : Inport
  Out1 : Outport
  wires:
  In1/1 -> Out1/1

== system example_sdofplant/actuator/fixed wing/actuator dyanmics/Variant Subsystem/Subsystem1 ==
  In1 : Inport
  Linear Second-Order Actuator : aerolibactuator/Linear Second-Order Actuator  wn_fin=1  z_fin=0.3  fin_act_0=0  fin_act_vel=0
  Out1 : Outport
  wires:
  Linear Second-Order Actuator/1 -> Out1/1
  In1/1 -> Linear Second-Order Actuator/1

== matlab function example_sdofplant/actuator/engine/Subsystem1/Dynamic_thrust ==
  data: rpm input; power input; thrust input; alt input; va input; rho input; blade_D input; thrust_d output
function thrust_d = dynamic_thrust(rpm, power, thrust, alt, va, rho, blade_D)

if power == 0
    thrust_d = 0;
else
    % 推力随着高度变化
    thrust_h = thrust * ((1-0.000022558 * alt)^4.2561 - 0.117)/0.883;
    % 推力随着速度变化
    thrust_d = thrust_h * (1-0.106 * 3.2808 * va * sqrt(rpm * (blade_D * 0.08333333)^3 /(power * 1.34 * 10 ^7 * (rho/1.225))));
end

== matlab function example_sdofplant/actuator/engine/Subsystem/Power_alt ==
  data: rho input; power_h output; power input
function power_h = power_by_alt(rho,power)
power_h = power * (rho/1.225-0.117)/0.883;
if power_h < 0
    power_h = 0;
end
